simulink model "drillingRigMss"  (R2015a)
settings: Solver=ode15s  StartTime=-1500  StopTime=1445  FixedStep=1e-3  RelTol=1e-6
values from neighbouring files (symbols this model uses):
  busTieOpens = 200    [initDrillingRigMSStoolbox.m]
  connectedGensets = [ones(1,engines-1) zeros(1,1)].'    [initDrillingRigMSStoolbox.m]
  connectedGensetsAfter = [ones(1,engines-2) zeros(1,2)].'    [initDrillingRigMSStoolbox.m]
  connectedGensetsSwitchTime = busTieOpens+50    (= 250)    [initDrillingRigMSStoolbox.m]
  connectedThrusters = [ones(1,nThrusters-0) zeros(1,0)].'    [initDrillingRigMSStoolbox.m]
  connectedThrustersAfter = [ones(1,nThrusters-1) zeros(1,1)].'    [initDrillingRigMSStoolbox.m]
  connectedThrustersSwitchTime = connectedGensetsSwitchTime+2    (= 252)    [initDrillingRigMSStoolbox.m]
  dAngleCost = 20    [initDrillingRigMSStoolbox.m]
  dfCost = 1    [initDrillingRigMSStoolbox.m]
  engines = 6    [initDrillingRigMSStoolbox.m]
  nSwitchboard = 3    [initDrillingRigMSStoolbox.m]
  nThrusters = 6    [initDrillingRigMSStoolbox.m]
  pmsSamplingTime = .1    (= 0.1)    [initDrillingRigMSStoolbox.m]
  rampTimeUpload = 30    [initDrillingRigMSStoolbox.m]
  singularityAvoidanceCostGain = .1    (= 0.1)    [initDrillingRigMSStoolbox.m]
  singularityAvoidanceCostSmoother = .0001    (= 0.0001)    [initDrillingRigMSStoolbox.m]
  thrustAllocationSamplingTime = 1    [initDrillingRigMSStoolbox.m]
  u_c = [-1 ... (first row only)    [initDrillingRigMSStoolbox.m]
  useObserver = 1    [initDrillingRigMSStoolbox.m]
  vNL0 = voltageNoQLoad*ones(engines,1)    [initDrillingRigMSStoolbox.m]
  waveForceAmplitude = 1*waveFrequency^2*.2*(vessel.MA(1,1)+vessel.MA(1,1))*[1;0;0]    [initDrillingRigMSStoolbox.m]
  waveFrequency = .3*2*pi    (= 1.88495559215)    [initDrillingRigMSStoolbox.m]
  windForce = D([1 2 6],[1 2 6])*u_c*1    [initDrillingRigMSStoolbox.m]
  wNL0 = 1./(1-Droop*.5)    [initDrillingRigMSStoolbox.m]
  x_ref = [0; 0; 0]    [initDrillingRigMSStoolbox.m]
undefined symbols (not defined in the file or in its folder): dp, generators, observer, TA_sampling_time, thrusters
undefined symbols (not defined in the file): vessel
libraries: genset x6, switchboard x6, thrusterLib x6, LoadOthers x3, simulink x2, pms x1, marine_gnc x1
settings Model: Creator=torstebo  LastModifiedBy=torstebo
settings SolverCC: SolverJacobianMethodControl=FullPerturbation
settings DataIOCC: Decimation=10  InitialState=xFinal  LimitDataPoints=off  LoadInitialState=on  SaveFinalState=on  SaveCompleteFinalSimState=on  SaveFormat=StructureWithTime  SaveOutput=off  DSMLogging=off  InspectSignalLogs=on  SaveTime=off
settings OptimizationCC: AccelVerboseBuild=on
settings DebuggingCC: UnderspecifiedInitializationDetection=Classic  MergeDetectMultiDrivingBlocksExec=none  SolverPrmCheckMsg=warning  StateNameClashWarn=warning

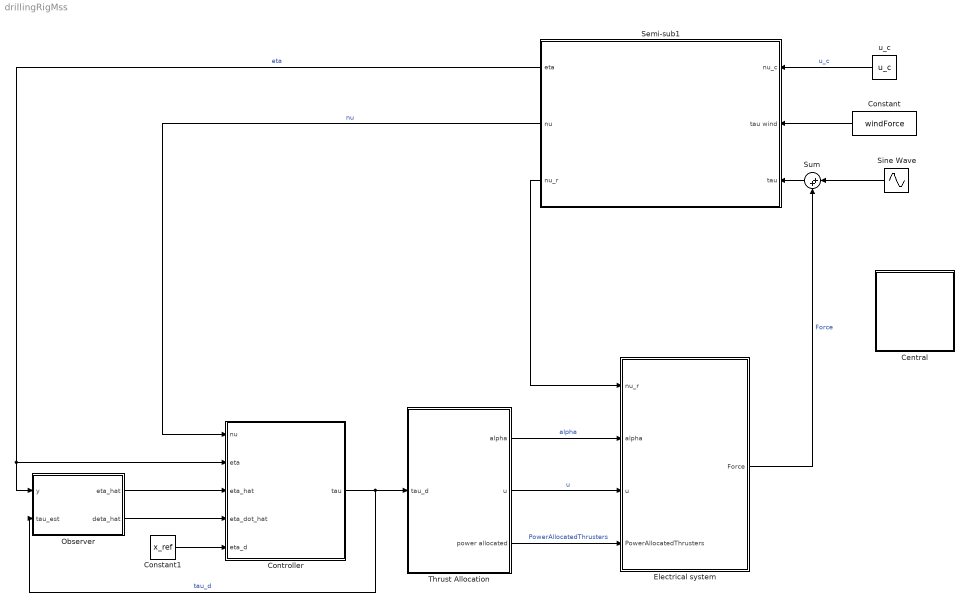
== system drillingRigMss ==
  Central : Subsystem
  Constant : Constant  Value=windForce
  Constant1 : Constant  Value=x_ref
  Controller : Subsystem
  Electrical system : Subsystem  Tag=electricSystem
  Observer : Subsystem
  Semi-sub1 : Subsystem  InitFcn=load MDGmodels/rig  mask(Semi-submersiblel (6 DOF)){D=vessel.D, G=vessel.G, MA=vessel.MA, MRB=vessel.MRB}
      mask prompts: D "Linear damping matrix: D"; G "Spring matrix G:"; MA "System inertia added mass matrix: M"; MRB "System inertia rigid-body matrix"
      mask help:
      | Semi-submersible low-speed model for DP.
      |
      | Inputs:
      |
      |    tau = 6 DOF control input vector (generalized force)
      |
      | Outputs:
      |
      |    eta = [x, y, z, phi, theta, psi]'
      |    nu  = [u, v, w, p, q, r]'
      mask Display:
      | image(imread('figs/semisub.jpg'))
      | color('white'); port_label('output', 1, 'eta')
      | color('white'); port_label('output', 2, 'nu')
      | color('white'); port_label('output', 3, 'nu_r')
      | color('white'); port_label('input', 1, 'nu_c')
      | color('white'); port_label('input', 2, 'tau wind')
      | color('white'); port_label('input', 3, 'tau')
  Sine Wave : Sin  Amplitude=waveForceAmplitude  Frequency=waveFrequency  SampleTime=0
  Sum : Sum  Inputs=|++
  Thrust Allocation : Subsystem  SystemSampleTime=TA_sampling_time
  u_c : Constant  Value=u_c
  wires:
  u_c/1 -> Semi-sub1/1(nu_c)  "u_c"
  Constant/1 -> Semi-sub1/2(tau wind)
  Semi-sub1/1(eta) -> Controller/2(eta), Observer/1(y)  "eta"
  Electrical system/1(Force) -> Sum/2  "Force"
  Controller/1(tau) -> Observer/2(tau_est), Thrust Allocation/1(tau_d)  "tau_d"
  Thrust Allocation/1(alpha) -> Electrical system/2(alpha)  "alpha"
  Thrust Allocation/2(u) -> Electrical system/3(u)  "u"
  Semi-sub1/3(nu_r) -> Electrical system/1(nu_r)
  Thrust Allocation/3(power allocated) -> Electrical system/4(PowerAllocatedThrusters)  "PowerAllocatedThrusters"
  Constant1/1 -> Controller/5(eta_d)
  Observer/2(deta_hat) -> Controller/4(eta_dot_hat)
  Observer/1(eta_hat) -> Controller/3(eta_hat)
  Sum/1 -> Semi-sub1/3(tau)
  Sine Wave/1 -> Sum/1
  Semi-sub1/2(nu) -> Controller/1(nu)  "nu"

== system drillingRigMss/Central ==
  Electric voltage calculations : Subsystem
  Event generator : Subsystem
  Power Management System : Subsystem  Tag=PowerManagementSystem

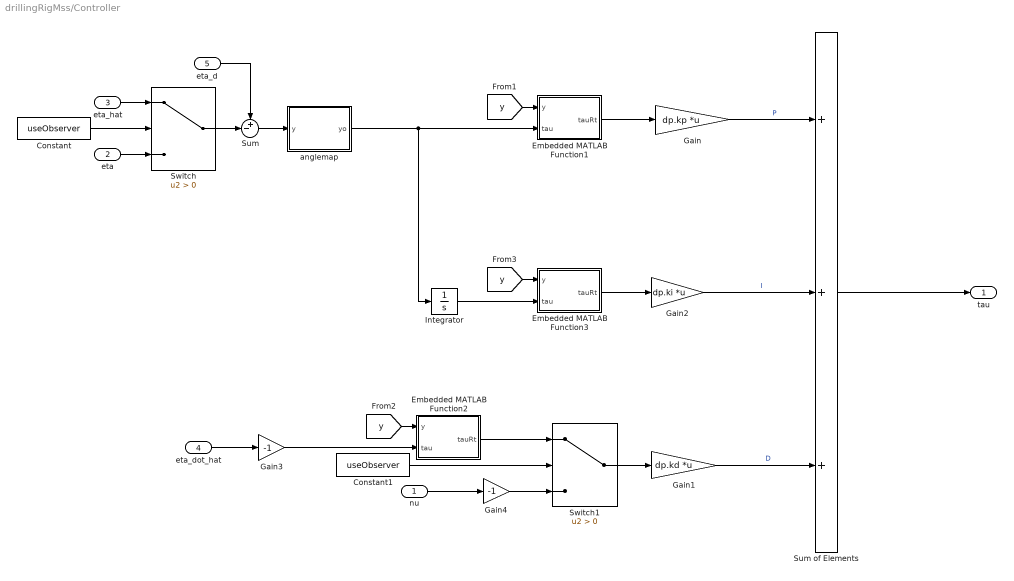
== system drillingRigMss/Controller ==
  nu : Inport
  eta : Inport  Port=2
  eta_hat : Inport  Port=3
  eta_dot_hat : Inport  Port=4
  eta_d : Inport  Port=5
  Constant : Constant  Value=useObserver
  Constant1 : Constant  Value=useObserver
  Embedded MATLAB Function1 : MATLAB Function  TreatAsAtomicUnit=on
  Embedded MATLAB Function2 : MATLAB Function  TreatAsAtomicUnit=on
  Embedded MATLAB Function3 : MATLAB Function  TreatAsAtomicUnit=on
  Gain : Gain  Gain=dp.kp  Multiplication=Matrix(K*u)
  Gain1 : Gain  Gain=dp.kd  Multiplication=Matrix(K*u)
  Gain2 : Gain  Gain=dp.ki  Multiplication=Matrix(K*u)
  Gain3 : Gain  Gain=-1
  Gain4 : Gain  Gain=-1
  Integrator : Integrator  InitialCondition=dp.ki\dp.tau0
  Sum : Sum  Inputs=+-|
  Sum of Elements : Sum  Inputs=3
  Switch : Switch  Criteria=u2 > Threshold
  Switch1 : Switch  Criteria=u2 > Threshold
  anglemap : MATLAB Function  TreatAsAtomicUnit=on
  tau : Outport
  wires:
  eta_d/1 -> Sum/1
  Gain1/1 -> Sum of Elements/3  "D"
  Sum of Elements/1 -> tau/1
  Sum/1 -> anglemap/1(y)
  [y] -> Embedded MATLAB Function1/1(y)
  Embedded MATLAB Function1/1(tauRt) -> Gain/1
  [y] -> Embedded MATLAB Function2/1(y)
  eta_dot_hat/1 -> Gain3/1
  Switch1/1 -> Gain1/1
  [y] -> Embedded MATLAB Function3/1(y)
  Integrator/1 -> Embedded MATLAB Function3/2(tau)
  Embedded MATLAB Function3/1(tauRt) -> Gain2/1
  Gain2/1 -> Sum of Elements/2  "I"
  Gain/1 -> Sum of Elements/1  "P"
  anglemap/1(yo) -> Embedded MATLAB Function1/2(tau), Integrator/1
  Gain3/1 -> Embedded MATLAB Function2/2(tau)
  nu/1 -> Gain4/1
  eta/1 -> Switch/3
  eta_hat/1 -> Switch/1
  Switch/1 -> Sum/2
  Constant/1 -> Switch/2
  Constant1/1 -> Switch1/2
  Embedded MATLAB Function2/1(tauRt) -> Switch1/1
  Gain4/1 -> Switch1/3

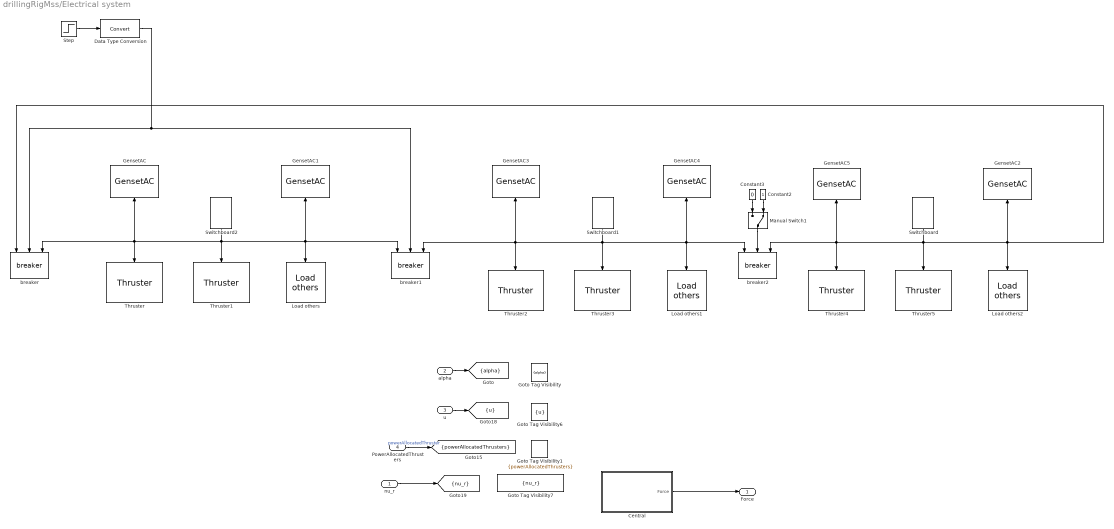
== system drillingRigMss/Electrical system ==
  nu_r : Inport  OutDataTypeStr=double
  alpha : Inport  Port=2  OutDataTypeStr=double
  u : Inport  Port=3  OutDataTypeStr=double
  PowerAllocatedThrusters : Inport  Port=4
  Central : Subsystem
  Constant2 : Constant  OutDataTypeStr=boolean
  Constant3 : Constant  Value=0  OutDataTypeStr=boolean
  Data Type Conversion : DataTypeConversion
  GensetAC : genset/GensetAC  Tag=GensetAC  genset=generators(1)  swbId=1
  GensetAC1 : genset/GensetAC  Tag=GensetAC  genset=generators(2)  swbId=1
  GensetAC2 : genset/GensetAC  Tag=GensetAC  genset=generators(6)  swbId=3
  GensetAC3 : genset/GensetAC  Tag=GensetAC  genset=generators(3)  swbId=2
  GensetAC4 : genset/GensetAC  Tag=GensetAC  genset=generators(4)  swbId=2
  GensetAC5 : genset/GensetAC  Tag=GensetAC  genset=generators(5)  swbId=3
  Goto Tag Visibility : GotoTagVisibility  GotoTag=alpha
  Goto Tag Visibility1 : GotoTagVisibility  GotoTag=powerAllocatedThrusters
  Goto Tag Visibility6 : GotoTagVisibility  GotoTag=u
  Goto Tag Visibility7 : GotoTagVisibility  GotoTag=nu_r
  Load others : LoadOthers/Load others  Tag=Load Others  swbId=1
  Load others1 : LoadOthers/Load others  Tag=Load Others  swbId=2
  Load others2 : LoadOthers/Load others  Tag=Load Others  swbId=3
  Manual Switch1 : ManualSwitch  CurrentSetting=0
  Step : Step  Time=busTieOpens  Before=1  After=0  SampleTime=0
  Switchboard : switchboard/Switchboard  Tag=Switchboard  swbId=3
  Switchboard1 : switchboard/Switchboard  Tag=Switchboard  swbId=2
  Switchboard2 : switchboard/Switchboard  Tag=Switchboard  swbId=1
  Thruster : thrusterLib/Thruster  Tag=Thruster  thruster=thrusters(1)  SwbId=1
      settings: AttributesFormatString=%<thruster>
  Thruster1 : thrusterLib/Thruster  Tag=Thruster  thruster=thrusters(2)  SwbId=1
      settings: AttributesFormatString=%<thruster>
  Thruster2 : thrusterLib/Thruster  Tag=Thruster  thruster=thrusters(3)  SwbId=2
      settings: AttributesFormatString=Thruster %<thruster.ID>
  Thruster3 : thrusterLib/Thruster  Tag=Thruster  thruster=thrusters(4)  SwbId=2
      settings: AttributesFormatString=Thruster %<thruster.ID>
  Thruster4 : thrusterLib/Thruster  Tag=Thruster  thruster=thrusters(5)  SwbId=3
      settings: AttributesFormatString=Thruster %<thruster.ID>
  Thruster5 : thrusterLib/Thruster  Tag=Thruster  thruster=thrusters(6)  SwbId=3
      settings: AttributesFormatString=Thruster %<thruster.ID>
  breaker : switchboard/breaker  Tag=SwitchboardBreaker  id=1
  breaker1 : switchboard/breaker  Tag=SwitchboardBreaker  id=2
  breaker2 : switchboard/breaker  Tag=SwitchboardBreaker  id=3
  Force : Outport  OutDataTypeStr=double
  tag scope: alpha=scoped, nu_r=scoped, powerAllocatedThrusters=scoped, u=scoped
  wires:
  alpha/1 -> [alpha]
  u/1 -> [u]
  nu_r/1 -> [nu_r]
  PowerAllocatedThrusters/1 -> [powerAllocatedThrusters]  "powerAllocatedThruster"
  Switchboard1/1 -> Thruster3/1, GensetAC4/1, breaker2/1, Load others1/1, GensetAC3/1, breaker1/3, Thruster2/1
  Switchboard/1 -> Thruster5/1, GensetAC2/1, breaker/1, Load others2/1, GensetAC5/1, breaker2/3, Thruster4/1
  Manual Switch1/1 -> breaker2/2
  Central/1(Force) -> Force/1
  Switchboard2/1 -> Thruster1/1, GensetAC/1, breaker/3, Thruster/1, GensetAC1/1, breaker1/1, Load others/1
  Constant2/1 -> Manual Switch1/2
  Constant3/1 -> Manual Switch1/1
  Data Type Conversion/1 -> breaker/2, breaker1/2
  Step/1 -> Data Type Conversion/1

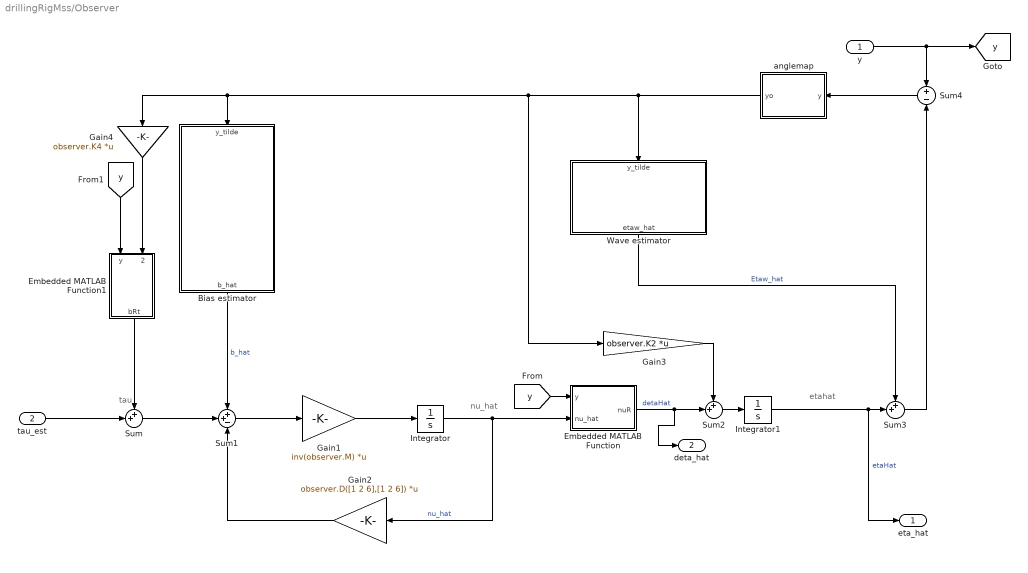
== system drillingRigMss/Observer ==
  note: nu_hat
  note: tau
  note: etahat
  y : Inport
  tau_est : Inport  Port=2
  Bias estimator : Subsystem
  Embedded MATLAB Function : MATLAB Function  TreatAsAtomicUnit=on
  Embedded MATLAB Function1 : MATLAB Function  TreatAsAtomicUnit=on
  Gain1 : Gain  Gain=inv(observer.M)  Multiplication=Matrix(K*u)
  Gain2 : Gain  Gain=observer.D([1 2 6],[1 2 6])  Multiplication=Matrix(K*u)
  Gain3 : Gain  Gain=observer.K2  Multiplication=Matrix(K*u)
  Gain4 : Gain  Gain=observer.K4  Multiplication=Matrix(K*u)
  Integrator : Integrator  InitialCondition=observer.nuHat0
  Integrator1 : Integrator  InitialCondition=observer.etaHat0
  Sum : Sum  Inputs=++|
  Sum1 : Sum  Inputs=++-
  Sum2 : Sum  Inputs=++|
  Sum3 : Sum  Inputs=++|
  Sum4 : Sum  Inputs=+-
  Wave estimator : Subsystem
  anglemap : MATLAB Function  TreatAsAtomicUnit=on
  eta_hat : Outport
  deta_hat : Outport  Port=2
  tag scope: y=global
  wires:
  tau_est/1 -> Sum/2
  Sum/1 -> Sum1/2
  Sum1/1 -> Gain1/1
  Gain1/1 -> Integrator/1
  Integrator/1 -> Gain2/1, Embedded MATLAB Function/2(nu_hat)  "nu_hat"
  Gain2/1 -> Sum1/3
  Embedded MATLAB Function/1(nuR) -> Sum2/2, deta_hat/1  "detaHat"
  Sum2/1 -> Integrator1/1
  Integrator1/1 -> Sum3/2, eta_hat/1  "etaHat"
  Sum3/1 -> Sum4/2
  y/1 -> Sum4/1, [y]
  Wave estimator/1(etaw_hat) -> Sum3/1  "Etaw_hat"
  Gain3/1 -> Sum2/1
  [y] -> Embedded MATLAB Function/1(y)
  Bias estimator/1(b_hat) -> Sum1/1  "b_hat"
  Gain4/1 -> Embedded MATLAB Function1/2(b_hat)
  [y] -> Embedded MATLAB Function1/1(y)
  Embedded MATLAB Function1/1(bRt) -> Sum/1
  Sum4/1 -> anglemap/1(y)
  anglemap/1(yo) -> Wave estimator/1(y_tilde), Gain3/1, Bias estimator/1(y_tilde), Gain4/1

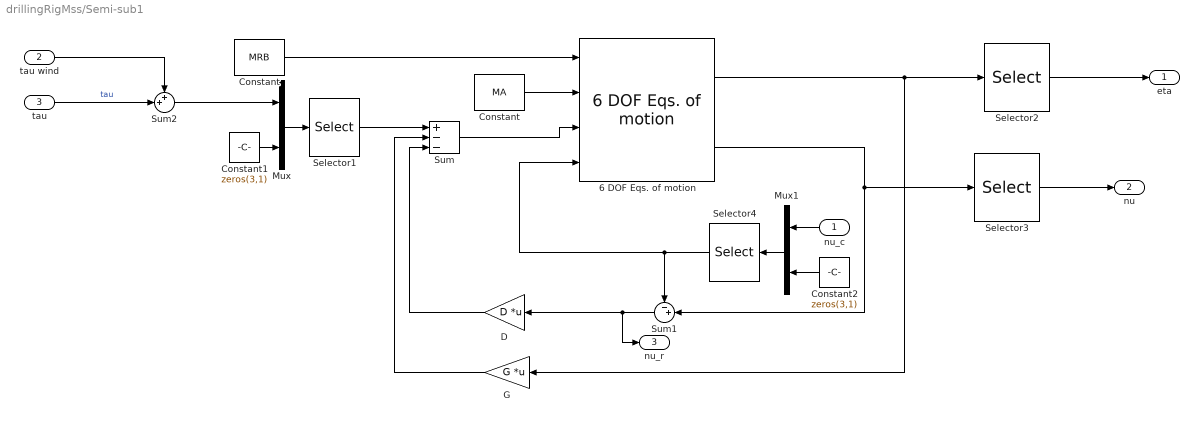
== system drillingRigMss/Semi-sub1 ==
  nu_c : Inport
  tau wind : Inport  Port=2
  tau : Inport  Port=3
  6 DOF Eqs. of motion : marine_gnc/Models/ Kinetics /6 DOF Eqs. of motion  CoriolisOnOff=on  nu0=vessel.nu0  eta0=vessel.eta0
  Constant : Constant  Value=MRB
  "Constant " : Constant  Value=MA
  Constant1 : Constant  Value=zeros(3,1)
  Constant2 : Constant  Value=zeros(3,1)
  D : Gain  Gain=D  Multiplication=Matrix(K*u)  SaturateOnIntegerOverflow=on  OutDataTypeStr=Inherit: Same as input  ParamDataTypeStr=Inherit: Same as input
  G : Gain  Gain=G  Multiplication=Matrix(K*u)  SaturateOnIntegerOverflow=on  OutDataTypeStr=Inherit: Same as input  ParamDataTypeStr=Inherit: Same as input
  Mux : Mux  Inputs=2
  Mux1 : Mux  Inputs=2
  Selector1 : Selector  InputPortWidth=6  Indices=[1 2 4 5 6 3]
  Selector2 : Selector  InputPortWidth=6  Indices=[1 2 6]
  Selector3 : Selector  InputPortWidth=6  Indices=[1 2 6]
  Selector4 : Selector  InputPortWidth=6  Indices=[1 2 4 5 6 3]
  Sum : Sum  Inputs=+--  SaturateOnIntegerOverflow=on  InputSameDT=on  OutDataTypeStr=Inherit: Same as first input
  Sum1 : Sum  Inputs=-+|  SaturateOnIntegerOverflow=on
  Sum2 : Sum  Inputs=++|
  eta : Outport  InitialOutput=0
  nu : Outport  Port=2  InitialOutput=0
  nu_r : Outport  Port=3  InitialOutput=0
  wires:
  D/1 -> Sum/3
  G/1 -> Sum/2
  6 DOF Eqs. of motion/2 -> Selector3/1, Sum1/2
  6 DOF Eqs. of motion/1 -> G/1, Selector2/1
  Constant/1 -> 6 DOF Eqs. of motion/1
  Selector4/1 -> Sum1/1, 6 DOF Eqs. of motion/4
  Sum1/1 -> nu_r/1, D/1
  Sum/1 -> 6 DOF Eqs. of motion/3
  "Constant "/1 -> 6 DOF Eqs. of motion/2
  Mux/1 -> Selector1/1
  Constant1/1 -> Mux/2
  tau/1 -> Sum2/2  "tau"
  tau wind/1 -> Sum2/1
  Sum2/1 -> Mux/1
  Selector1/1 -> Sum/1
  Selector2/1 -> eta/1
  Selector3/1 -> nu/1
  Mux1/1 -> Selector4/1
  Constant2/1 -> Mux1/2
  nu_c/1 -> Mux1/1

== system drillingRigMss/Thrust Allocation ==
  tau_d : Inport
  Constant : Constant  Value=-1
  Constant1 : Constant  Value=-1
  For Each Subsystem1 : Subsystem  TreatAsAtomicUnit=on
  From Thrusters : Subsystem  Tag=ThrusterAllocation/FromThrusters
  Subsystem : Subsystem
  Sum : Sum  Inputs=|++
  Sum1 : Sum  Inputs=|++
  Zero-Order Hold : ZeroOrderHold  SampleTime=thrustAllocationSamplingTime
  alpha : Outport
  u : Outport  Port=2
  power allocated : Outport  Port=3
  wires:
  For Each Subsystem1/11(turnTime) -> Subsystem/16(turnTime)  "turnTime"
  For Each Subsystem1/7(KT2P) -> Subsystem/12(KT2P)  "KT2P"
  For Each Subsystem1/6(Thrusters on) -> Subsystem/11(Thrusters on)  "thurstersOn"
  For Each Subsystem1/5(u_old) -> Subsystem/10(f_old)  "f"
  For Each Subsystem1/4(alpha) -> Subsystem/9(Alpha_old)  "alpha"
  For Each Subsystem1/3(Tau Max) -> Subsystem/8(Tau Max)  "tauMax"
  For Each Subsystem1/2(ThrusterPostitionY) -> Subsystem/7(Thruster Position Y)  "posY"
  For Each Subsystem1/1(ThrusterPostitionX) -> Subsystem/6(Thruster Position X)  "posX"
  [nBus] -> Subsystem/5(N bus)  "nBus"
  Sum/1 -> Subsystem/4(Switchboard to bus)  "s2b"
  tau_d/1 -> Subsystem/1(tau_d)  "tau_d"
  Constant/1 -> Sum/2
  [switchboard2bus] -> Sum/1
  From Thrusters/1(Thruster) -> Zero-Order Hold/1  "Thruster"
  Sum1/1 -> Subsystem/13(Thruster 2 Switchboard)  "t2s"
  Constant1/1 -> Sum1/2
  For Each Subsystem1/8(Thruster 2 Switchboard) -> Sum1/1
  For Each Subsystem1/9(fRampTime) -> Subsystem/14(fRampTime)  "fRampTime"
  For Each Subsystem1/10(f min) -> Subsystem/15(u min)  "fMin"
  For Each Subsystem1/12(rotable) -> Subsystem/17(rotable)  "rotable"
  For Each Subsystem1/13(reversePowerFactor) -> Subsystem/18(Reverse thrust power gain)  "reversePowerFactor"
  [FastLoadReductionThrusters] -> Subsystem/3(Fast Load Reduction Thruster)  "FLR"
  Zero-Order Hold/1 -> For Each Subsystem1/1(In1)
  [powerAvailableDP] -> Subsystem/2(Power Available Bus)  "pADP"
  Subsystem/2(U) -> u/1  "u"
  Subsystem/3(Power Allocated) -> power allocated/1
  Subsystem/1(Alpha) -> alpha/1  "alpha"

== system drillingRigMss/Central/Electric voltage calculations ==
  Busses : Subsystem
      mask Display:
      | image(imread('figs/switchboard.jpg'))
      | port_label('input',1,'Power Loads')
      | port_label('input',2,'nbus')
      | port_label('input',3,'switchboard2bus')
      | port_label('input',4,'Generators')
      | port_label('output',1,'switchboard')
  From Gensets : Subsystem  Tag=FromGeneratorsetElectric
  From breakers : Subsystem  Tag=FromBreakers
  From loads : Subsystem  Tag=FromLoads
  Switchboard2Bus : Subsystem  Tag=Switchboard2Bus  mask{nSwitchboards=3}
      mask prompts: nSwitchboards "Number of Switchboards"
  tag scope: switchboard=global
  wires:
  From breakers/1(Breakers) -> Switchboard2Bus/1(Breakers)
  From loads/1(Loads) -> Busses/1(powerLoads)
  From Gensets/1(Generators) -> Busses/4(Generatorset)
  Switchboard2Bus/2(switchboard2bus) -> Busses/3(switchboard2bus)
  Switchboard2Bus/1(nbus) -> Busses/2(nbus)
  Busses/1(switchboard bus) -> [switchboard]

== system drillingRigMss/Central/Event generator ==
  Compare To Constant : simulink/Logic and Bit Operations/Compare To Constant  relop=>  const=0  OutDataTypeStr=boolean
  Compare To Constant1 : simulink/Logic and Bit Operations/Compare To Constant  relop=>  const=0  OutDataTypeStr=boolean
  Step1 : Step  Time=connectedGensetsSwitchTime  Before=connectedGensets  After=connectedGensetsAfter  SampleTime=0
  Step2 : Step  Time=connectedThrustersSwitchTime  Before=connectedThrusters  After=connectedThrustersAfter  SampleTime=0
  tag scope: gensetsOn=global, thrustersOn=global
  wires:
  Compare To Constant1/1 -> [thrustersOn]
  Step1/1 -> Compare To Constant/1
  Compare To Constant/1 -> [gensetsOn]
  Step2/1 -> Compare To Constant1/1

== system drillingRigMss/Central/Power Management System ==
  From Batteries : Subsystem  Tag=PowerManagementSystem/FromBatteries  Commented=on
  From Generatorsets : Subsystem  Tag=PowerManagementSystem/FromGeneratorset
  From Load others : Subsystem  Tag=PowerManagementSystem/LoadOthersFrom
  From Thrusters : Subsystem  Tag=PowerManagementSystem/ThrusterFrom
  Genset Control : Subsystem
  Log Power : Subsystem
  Power Management System : pms/Subsystem  TSample=pmsSamplingTime  reactionTimePowerAvaialble=reactionTimePowerAvaialble  rampTimePowerAvaialble=rampTimePowerAvaialble  FlrRestoreTime=flrRestoreTime  FlrRampTime=flrRampTime  nSwb=nSwitchboard  nThruster=nThrusters  nBatteries=nBatteries  DPPowerAvailableBias=powerDesiredDPBias  DPPowerAvailableGain=powerDesiredDPGain  PMSenableFaultDetection=PMSenableFaultDetection
  Terminator : Terminator
  Terminator2 : Terminator
  tag scope: FastLoadReductionThrusters=global, GensetVNL=global, GensetWNL=global, powerAvailableDP=global, powerAvailableHighPriority=global, powerAvailableLowPriority=global
  wires:
  Power Management System/4 -> Log Power/2(FastLoadReductionThrusters), [FastLoadReductionThrusters]  "PowerAvailableThrusters"
  Power Management System/6 -> Log Power/4(powerAvailableHighPriority), [powerAvailableHighPriority]  "PowerAvailableHP"
  Power Management System/3 -> Log Power/1(powerAvailableDP), [powerAvailableDP]  "powerAvailableDP"
  Power Management System/5 -> Log Power/3(powerAvailableLowPriority), [powerAvailableLowPriority]  "PowerAvailableLP"
  [nBus] -> Power Management System/2
  Power Management System/1 -> Terminator2/1  "powerDP"
  Power Management System/2 -> Terminator/1  "powerDesiredDP"
  [switchboard2bus] -> Power Management System/1
  From Load others/1(PowerDesiredLowPriority) -> Power Management System/3
  From Load others/3(PowerDesiredHighPriority) -> Power Management System/5
  From Load others/2(PowerLowPriority) -> Power Management System/4
  From Load others/4(PowerHighPriority) -> Power Management System/6
  From Thrusters/1(Thruster Power) -> Power Management System/7
  From Thrusters/2(Thruster2SwbId) -> Power Management System/8
  From Thrusters/3(Thruster RatedPower) -> Power Management System/9
  From Thrusters/4(Thruster Connected) -> Power Management System/10
  From Generatorsets/1(GensetsDeliveredPower) -> Power Management System/14
  From Generatorsets/2(GensetsPowerAvailable) -> Power Management System/15
  From Generatorsets/4(GensetsRatedPower) -> Power Management System/17
  Genset Control/1(wNL) -> [GensetWNL]
  From Generatorsets/3(GensetsConnected) -> Power Management System/16
  From Generatorsets/5(GensetsSwbID) -> Genset Control/1(GensetsSwbID), Power Management System/18
  From Generatorsets/6(GensetsConnected1) -> Genset Control/2(GensetsConnected)
  Genset Control/2(vNL) -> [GensetVNL]
  From Batteries/3(BatteriesSwbId) -> Power Management System/13
  From Batteries/2(BatteriesPowerAvailable) -> Power Management System/12
  From Batteries/1(BatteriesDeliveredPower) -> Power Management System/11

== system drillingRigMss/Electrical system/Central ==
  From Force : Subsystem  Tag=ForceFrom
  Force : Outport  Tag=ForceFrom  OutDataTypeStr=double
  wires:
  From Force/1(Force) -> Force/1

== system drillingRigMss/Observer/Bias estimator ==
  y_tilde : Inport
  Embedded MATLAB Function : MATLAB Function  TreatAsAtomicUnit=on
  Gain3 : Gain  Gain=observer.K3  Multiplication=Matrix(K*u)
  Gain4 : Gain  Gain=inv(observer.T)  Multiplication=Matrix(K*u)
  Integrator1 : Integrator  InitialCondition=observer.biasForce0
  Sum1 : Sum  Inputs=+-
  b_hat : Outport
  wires:
  y_tilde/1 -> Gain3/1
  Gain3/1 -> Sum1/1
  Sum1/1 -> Integrator1/1
  Gain4/1 -> Sum1/2
  Integrator1/1 -> Gain4/1, Embedded MATLAB Function/2(b_hat)
  Embedded MATLAB Function/1(bRt) -> b_hat/1
  [y] -> Embedded MATLAB Function/1(y)

== system drillingRigMss/Observer/Wave estimator ==
  y_tilde : Inport
  Gain1 : Gain  Gain=observer.Aw  Multiplication=Matrix(K*u)
  Gain2 : Gain  Gain=observer.Cw  Multiplication=Matrix(K*u)
  Gain3 : Gain  Gain=observer.K1  Multiplication=Matrix(K*u)
  Integrator : Integrator  InitialCondition=[0 0 0 0 0 0]'
  Sum : Sum  Inputs=|++
  etaw_hat : Outport  PortDimensions=3
  wires:
  y_tilde/1 -> Gain3/1
  Gain3/1 -> Sum/1
  Sum/1 -> Integrator/1
  Integrator/1 -> Gain1/1, Gain2/1
  Gain1/1 -> Sum/2
  Gain2/1 -> etaw_hat/1

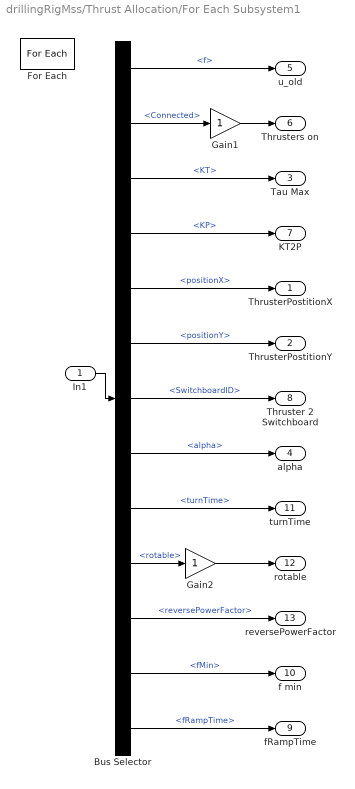
== system drillingRigMss/Thrust Allocation/For Each Subsystem1 ==
  In1 : Inport  OutDataTypeStr=Bus: ThrusterBus  Partition=on  PartitionDimension=1  PartitionWidth=1
  Bus Selector : BusSelector  OutputSignals=f,Connected,KT,KP,positionX,positionY,SwitchboardID,alpha,turnTime,rotable,reversePowerFactor,fMin,fRampTime
  For Each : ForEach  DisableCoverage=on  IndexMode=One-based
  Gain1 : Gain  OutDataTypeStr=double
  Gain2 : Gain  OutDataTypeStr=double
  ThrusterPostitionX : Outport  ConcatenationDimension=1
  ThrusterPostitionY : Outport  Port=2  ConcatenationDimension=1
  Tau Max : Outport  Port=3  ConcatenationDimension=1
  alpha : Outport  Port=4  ConcatenationDimension=1
  u_old : Outport  Port=5  ConcatenationDimension=1
  Thrusters on : Outport  Port=6  ConcatenationDimension=1
  KT2P : Outport  Port=7  ConcatenationDimension=1
  Thruster 2 Switchboard : Outport  Port=8  ConcatenationDimension=1
  fRampTime : Outport  Port=9  ConcatenationDimension=1
  f min : Outport  Port=10  ConcatenationDimension=1
  turnTime : Outport  Port=11  ConcatenationDimension=1
  rotable : Outport  Port=12  ConcatenationDimension=1
  reversePowerFactor : Outport  Port=13  ConcatenationDimension=1
  wires:
  Bus Selector/13 -> fRampTime/1  "<fRampTime>"
  Bus Selector/12 -> f min/1  "<fMin>"
  Bus Selector/11 -> reversePowerFactor/1  "<reversePowerFactor>"
  Bus Selector/9 -> turnTime/1  "<turnTime>"
  Bus Selector/10 -> Gain2/1  "<rotable>"
  Bus Selector/8 -> alpha/1  "<alpha>"
  Bus Selector/7 -> Thruster 2 Switchboard/1  "<SwitchboardID>"
  Bus Selector/6 -> ThrusterPostitionY/1  "<positionY>"
  Bus Selector/5 -> ThrusterPostitionX/1  "<positionX>"
  Gain1/1 -> Thrusters on/1
  Bus Selector/4 -> KT2P/1  "<KP>"
  Bus Selector/3 -> Tau Max/1  "<KT>"
  Bus Selector/2 -> Gain1/1  "<Connected>"
  Bus Selector/1 -> u_old/1  "<f>"
  In1/1 -> Bus Selector/1
  Gain2/1 -> rotable/1

== system drillingRigMss/Thrust Allocation/From Thrusters ==
  Vector Concatenate : Concatenate  Tag=FromThrusters/Merger  NumInputs=6
  Thruster : Outport
  wires:
  Vector Concatenate/1 -> Thruster/1
  [Thruster1] -> Vector Concatenate/1
  [Thruster2] -> Vector Concatenate/2
  [Thruster3] -> Vector Concatenate/3
  [Thruster4] -> Vector Concatenate/4
  [Thruster5] -> Vector Concatenate/5
  [Thruster6] -> Vector Concatenate/6

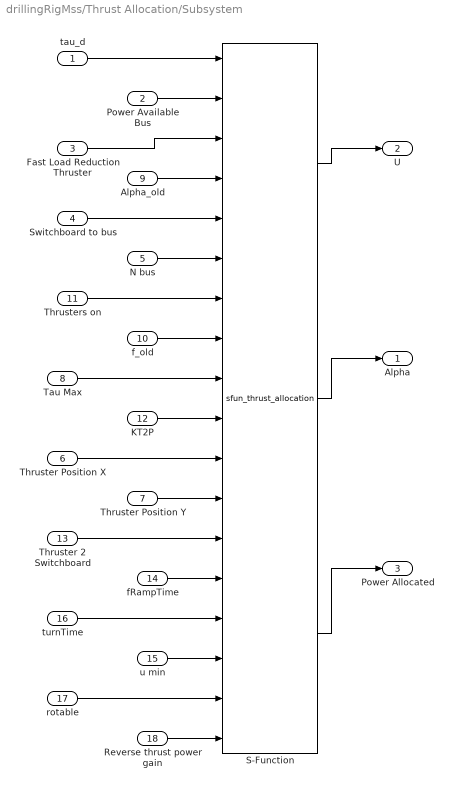
== system drillingRigMss/Thrust Allocation/Subsystem ==
  tau_d : Inport
  Power Available Bus : Inport  Port=2
  Fast Load Reduction Thruster : Inport  Port=3
  Switchboard to bus : Inport  Port=4
  N bus : Inport  Port=5
  Thruster Position X : Inport  Port=6
  Thruster Position Y : Inport  Port=7
  Tau Max : Inport  Port=8
  Alpha_old : Inport  Port=9
  f_old : Inport  Port=10
  Thrusters on : Inport  Port=11
  KT2P : Inport  Port=12
  Thruster 2 Switchboard : Inport  Port=13
  fRampTime : Inport  Port=14
  u min : Inport  Port=15
  turnTime : Inport  Port=16
  rotable : Inport  Port=17
  Reverse thrust power gain : Inport  Port=18
  S-Function : S-Function  FunctionName=sfun_thrust_allocation  Parameters=thrustAllocationSamplingTime,nThrusters,nSwitchboard,singularityAvoidanceCostGain,singularityAvoidanceCostSmoother,dfCost,dAngleCost
  Alpha : Outport
  U : Outport  Port=2
  Power Allocated : Outport  Port=3
  wires:
  f_old/1 -> S-Function/8
  Thrusters on/1 -> S-Function/7
  N bus/1 -> S-Function/6
  Switchboard to bus/1 -> S-Function/5
  Alpha_old/1 -> S-Function/4
  Fast Load Reduction Thruster/1 -> S-Function/3
  tau_d/1 -> S-Function/1
  Power Available Bus/1 -> S-Function/2
  S-Function/1 -> U/1
  S-Function/2 -> Alpha/1
  turnTime/1 -> S-Function/15
  fRampTime/1 -> S-Function/14
  Thruster 2 Switchboard/1 -> S-Function/13
  Thruster Position Y/1 -> S-Function/12
  Thruster Position X/1 -> S-Function/11
  KT2P/1 -> S-Function/10
  Tau Max/1 -> S-Function/9
  u min/1 -> S-Function/16
  S-Function/3 -> Power Allocated/1
  rotable/1 -> S-Function/17
  Reverse thrust power gain/1 -> S-Function/18

== system drillingRigMss/Central/Electric voltage calculations/Busses ==
  powerLoads : Inport  OutDataTypeStr=Bus: powerLoadsBus
  nbus : Inport  Port=2
  switchboard2bus : Inport  Port=3
  Generatorset : Inport  Port=4
  Constant2 : Constant  Value=-1
  Integrator : Integrator
  MATLAB Function1 : MATLAB Function  TreatAsAtomicUnit=on
  Merge loads : MATLAB Function  TreatAsAtomicUnit=on
  Saturation : Saturate  UpperLimit=0  LowerLimit=-1
  Sum : Sum  Inputs=++|
  Switchboard1 : MATLAB Function  TreatAsAtomicUnit=on
  Thevenin Equivalent : MATLAB Function  TreatAsAtomicUnit=on
  switchboard bus : Outport
  wires:
  Switchboard1/1(out) -> switchboard bus/1
  powerLoads/1 -> Merge loads/1(load)  "power bus"
  switchboard2bus/1 -> Switchboard1/2(switchboard2bus), Merge loads/2(swb2bus), Thevenin Equivalent/2(switchboard2bus)  "s2b"
  Generatorset/1 -> Thevenin Equivalent/3(generatorset)  "Generatorset"
  Integrator/1 -> MATLAB Function1/1(u)
  Constant2/1 -> Sum/1
  Sum/1 -> Saturation/1
  Switchboard1/2(isInputValid) -> Sum/2
  nbus/1 -> Switchboard1/3(nbus), Thevenin Equivalent/1(nbus)  "nbus"
  Merge loads/1(loads) -> Switchboard1/1(powerLoads)  "load"
  Thevenin Equivalent/1(theveninEquivalent) -> Switchboard1/4(generatorset)
  Saturation/1 -> Integrator/1

== system drillingRigMss/Central/Electric voltage calculations/From Gensets ==
  Merger : Concatenate  Tag=FromGeneratorsetElectric/Merger  NumInputs=6
  Generators : Outport
  wires:
  Merger/1 -> Generators/1
  [GeneratorsetElectric1] -> Merger/1
  [GeneratorsetElectric2] -> Merger/2
  [GeneratorsetElectric6] -> Merger/6
  [GeneratorsetElectric3] -> Merger/3
  [GeneratorsetElectric4] -> Merger/4
  [GeneratorsetElectric5] -> Merger/5

== system drillingRigMss/Central/Electric voltage calculations/From breakers ==
  MergerBreakers : Concatenate  Tag=FromBreakers/MergerBreakers  NumInputs=3
  Breakers : Outport
  wires:
  MergerBreakers/1 -> Breakers/1
  [Breaker1] -> MergerBreakers/1
  [Breaker2] -> MergerBreakers/2
  [Breaker3] -> MergerBreakers/3

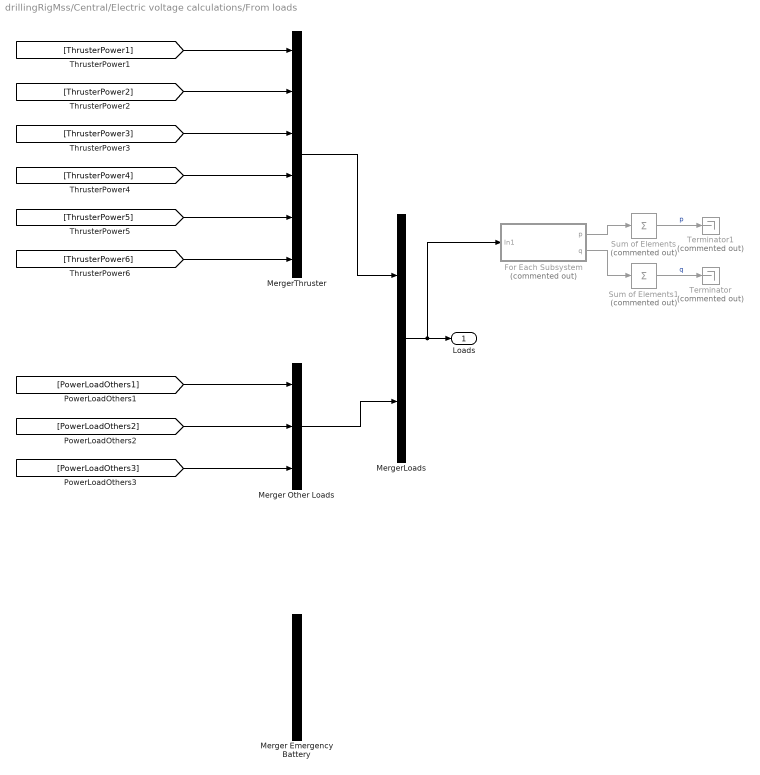
== system drillingRigMss/Central/Electric voltage calculations/From loads ==
  For Each Subsystem : Subsystem  Commented=on  TreatAsAtomicUnit=on
  Merger Emergency Battery : Concatenate  Tag=FromLoads/MergerEmergencyBattery  NumInputs=1
  Merger Other Loads : Concatenate  Tag=FromLoads/MergerOtherLoads  NumInputs=3
  MergerLoads : Concatenate  Tag=FromLoads/MergerLoads
  MergerThruster : Concatenate  Tag=FromLoads/MergerThruster  NumInputs=6
  Sum of Elements : Sum  Commented=on  Inputs=+
  Sum of Elements1 : Sum  Commented=on  Inputs=+
  Terminator : Terminator  Commented=on
  Terminator1 : Terminator  Commented=on
  Loads : Outport
  wires:
  MergerThruster/1 -> MergerLoads/1
  Merger Other Loads/1 -> MergerLoads/2
  MergerLoads/1 -> For Each Subsystem/1(In1), Loads/1
  For Each Subsystem/1(p) -> Sum of Elements/1
  For Each Subsystem/2(q) -> Sum of Elements1/1
  Sum of Elements1/1 -> Terminator/1  "q"
  Sum of Elements/1 -> Terminator1/1  "p"
  [PowerLoadOthers1] -> Merger Other Loads/1
  [PowerLoadOthers2] -> Merger Other Loads/2
  [PowerLoadOthers3] -> Merger Other Loads/3
  [ThrusterPower1] -> MergerThruster/1
  [ThrusterPower2] -> MergerThruster/2
  [ThrusterPower3] -> MergerThruster/3
  [ThrusterPower4] -> MergerThruster/4
  [ThrusterPower5] -> MergerThruster/5
  [ThrusterPower6] -> MergerThruster/6

== system drillingRigMss/Central/Electric voltage calculations/Switchboard2Bus ==
  Breakers : Inport
  MATLAB Function : MATLAB Function  TreatAsAtomicUnit=on
  nbus : Outport
  switchboard2bus : Outport  Port=2
  tag scope: nBus=global, switchboard2bus=global
  wires:
  MATLAB Function/2(switchboard2bus) -> switchboard2bus/1, [switchboard2bus]
  MATLAB Function/1(nbus) -> nbus/1, [nBus]
  Breakers/1 -> MATLAB Function/1(breaker)

== system drillingRigMss/Central/Power Management System/From Batteries ==
  For Each Subsystem : Subsystem  TreatAsAtomicUnit=on
  Vector Concatenate : Concatenate  Tag=PowerManagementSystem/FromBatteries/Merger  NumInputs=1
  Zero-Order Hold : ZeroOrderHold  SampleTime=pmsSamplingTime
  BatteriesDeliveredPower : Outport
  BatteriesPowerAvailable : Outport  Port=2
  BatteriesSwbId : Outport  Port=3
  wires:
  For Each Subsystem/3(switchboardId) -> BatteriesSwbId/1
  For Each Subsystem/2(powerAvailable) -> BatteriesPowerAvailable/1
  For Each Subsystem/1(powerDelivered) -> BatteriesDeliveredPower/1
  Vector Concatenate/1 -> Zero-Order Hold/1
  Zero-Order Hold/1 -> For Each Subsystem/1(In1)
  [EmergencyBattery1] -> Vector Concatenate/1

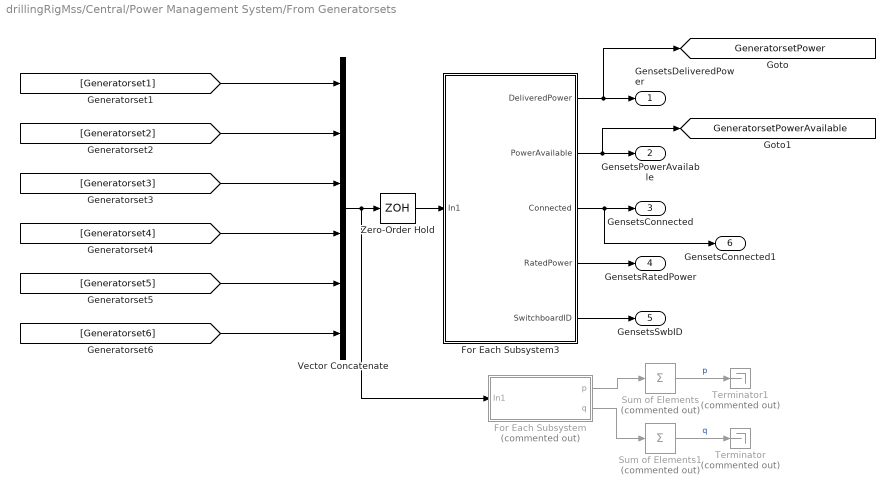
== system drillingRigMss/Central/Power Management System/From Generatorsets ==
  For Each Subsystem : Subsystem  Commented=on  TreatAsAtomicUnit=on
  For Each Subsystem3 : Subsystem  TreatAsAtomicUnit=on
  Sum of Elements : Sum  Commented=on  Inputs=+
  Sum of Elements1 : Sum  Commented=on  Inputs=+
  Terminator : Terminator  Commented=on
  Terminator1 : Terminator  Commented=on
  Vector Concatenate : Concatenate  Tag=PowerManagementSystem/FromGeneratorset/Merger  NumInputs=6
  Zero-Order Hold : ZeroOrderHold  SampleTime=pmsSamplingTime
  GensetsDeliveredPower : Outport  OutDataTypeStr=double
  GensetsPowerAvailable : Outport  Port=2  OutDataTypeStr=double
  GensetsConnected : Outport  Port=3  OutDataTypeStr=boolean
  GensetsRatedPower : Outport  Port=4  OutDataTypeStr=double
  GensetsSwbID : Outport  Port=5  OutDataTypeStr=uint8
  GensetsConnected1 : Outport  Port=6  OutDataTypeStr=boolean
  tag scope: GeneratorsetPower=global, GeneratorsetPowerAvailable=global
  wires:
  For Each Subsystem3/3(Connected) -> GensetsConnected1/1, GensetsConnected/1
  For Each Subsystem3/5(SwitchboardID) -> GensetsSwbID/1
  For Each Subsystem3/2(PowerAvailable) -> [GeneratorsetPowerAvailable], GensetsPowerAvailable/1
  For Each Subsystem3/4(RatedPower) -> GensetsRatedPower/1
  For Each Subsystem3/1(DeliveredPower) -> [GeneratorsetPower], GensetsDeliveredPower/1
  Vector Concatenate/1 -> Zero-Order Hold/1, For Each Subsystem/1(In1)
  For Each Subsystem/1(p) -> Sum of Elements/1
  For Each Subsystem/2(q) -> Sum of Elements1/1
  Sum of Elements1/1 -> Terminator/1  "q"
  Sum of Elements/1 -> Terminator1/1  "p"
  Zero-Order Hold/1 -> For Each Subsystem3/1(In1)
  [Generatorset1] -> Vector Concatenate/1
  [Generatorset2] -> Vector Concatenate/2
  [Generatorset6] -> Vector Concatenate/6
  [Generatorset3] -> Vector Concatenate/3
  [Generatorset4] -> Vector Concatenate/4
  [Generatorset5] -> Vector Concatenate/5

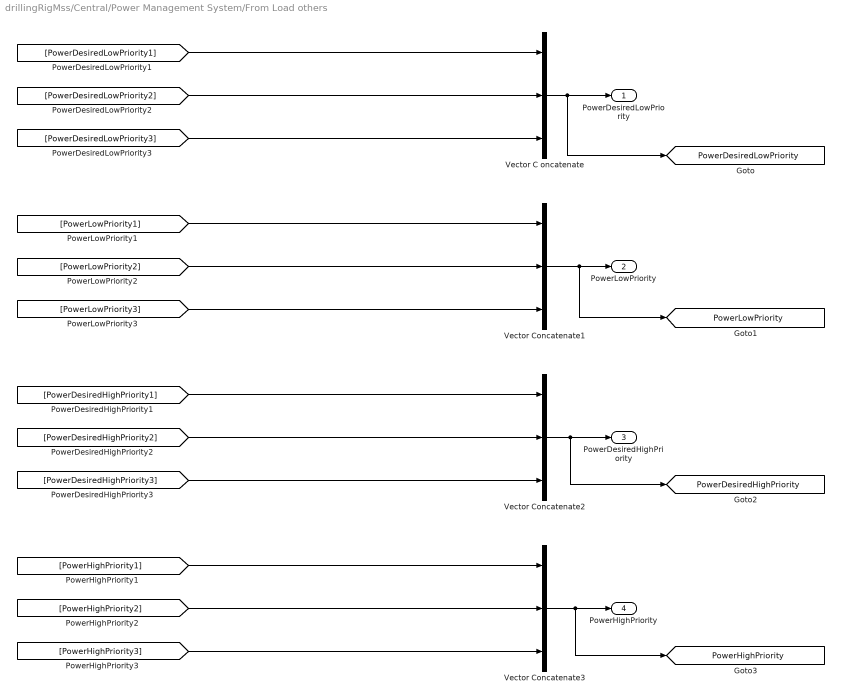
== system drillingRigMss/Central/Power Management System/From Load others ==
  Vector C oncatenate : Concatenate  Tag=PowerManagementSystem/LoadOthersFrom/PowerDesiredLowPriority  NumInputs=3
  Vector Concatenate1 : Concatenate  Tag=PowerManagementSystem/LoadOthersFrom/PowerLowPriority  NumInputs=3
  Vector Concatenate2 : Concatenate  Tag=PowerManagementSystem/LoadOthersFrom/PowerDesiredHighPriority  NumInputs=3
  Vector Concatenate3 : Concatenate  Tag=PowerManagementSystem/LoadOthersFrom/PowerHighPriority  NumInputs=3
  PowerDesiredLowPriority : Outport
  PowerLowPriority : Outport  Port=2
  PowerDesiredHighPriority : Outport  Port=3
  PowerHighPriority : Outport  Port=4
  tag scope: PowerDesiredHighPriority=global, PowerDesiredLowPriority=global, PowerHighPriority=global, PowerLowPriority=global
  wires:
  Vector C oncatenate/1 -> PowerDesiredLowPriority/1, [PowerDesiredLowPriority]
  Vector Concatenate1/1 -> [PowerLowPriority], PowerLowPriority/1
  Vector Concatenate2/1 -> [PowerDesiredHighPriority], PowerDesiredHighPriority/1
  Vector Concatenate3/1 -> [PowerHighPriority], PowerHighPriority/1
  [PowerDesiredLowPriority1] -> Vector C oncatenate/1
  [PowerLowPriority1] -> Vector Concatenate1/1
  [PowerDesiredHighPriority1] -> Vector Concatenate2/1
  [PowerHighPriority1] -> Vector Concatenate3/1
  [PowerDesiredLowPriority2] -> Vector C oncatenate/2
  [PowerLowPriority2] -> Vector Concatenate1/2
  [PowerDesiredHighPriority2] -> Vector Concatenate2/2
  [PowerHighPriority2] -> Vector Concatenate3/2
  [PowerDesiredLowPriority3] -> Vector C oncatenate/3
  [PowerLowPriority3] -> Vector Concatenate1/3
  [PowerDesiredHighPriority3] -> Vector Concatenate2/3
  [PowerHighPriority3] -> Vector Concatenate3/3

== system drillingRigMss/Central/Power Management System/From Thrusters ==
  For Each Subsystem : Subsystem  TreatAsAtomicUnit=on
  Vector Concatenate : Concatenate  Tag=FromThrusters/Merger  NumInputs=6
  Zero-Order Hold : ZeroOrderHold  SampleTime=pmsSamplingTime
  Thruster Power : Outport
  Thruster2SwbId : Outport  Port=2
  Thruster RatedPower : Outport  Port=3
  Thruster Connected : Outport  Port=4
  tag scope: ThrusterPower=global
  wires:
  For Each Subsystem/3(RatedPower) -> Thruster RatedPower/1
  For Each Subsystem/2(switchboardId) -> Thruster2SwbId/1
  For Each Subsystem/1(power) -> [ThrusterPower], Thruster Power/1
  For Each Subsystem/4(Connected) -> Thruster Connected/1
  Vector Concatenate/1 -> Zero-Order Hold/1
  Zero-Order Hold/1 -> For Each Subsystem/1(In1)
  [Thruster1] -> Vector Concatenate/1
  [Thruster2] -> Vector Concatenate/2
  [Thruster3] -> Vector Concatenate/3
  [Thruster4] -> Vector Concatenate/4
  [Thruster5] -> Vector Concatenate/5
  [Thruster6] -> Vector Concatenate/6

== system drillingRigMss/Central/Power Management System/Genset Control ==
  GensetsSwbID : Inport
  GensetsConnected : Inport  Port=2
  Clock : Clock
  MATLAB Function : MATLAB Function  TreatAsAtomicUnit=on
  wNL : Outport
  vNL : Outport  Port=2
  wires:
  MATLAB Function/1(wNL) -> wNL/1
  [switchboard] -> MATLAB Function/2(switchboard)
  GensetsConnected/1 -> MATLAB Function/1(gensetConnected)
  GensetsSwbID/1 -> MATLAB Function/3(gensetSwbId)
  Clock/1 -> MATLAB Function/4(time)
  MATLAB Function/2(vNL) -> vNL/1

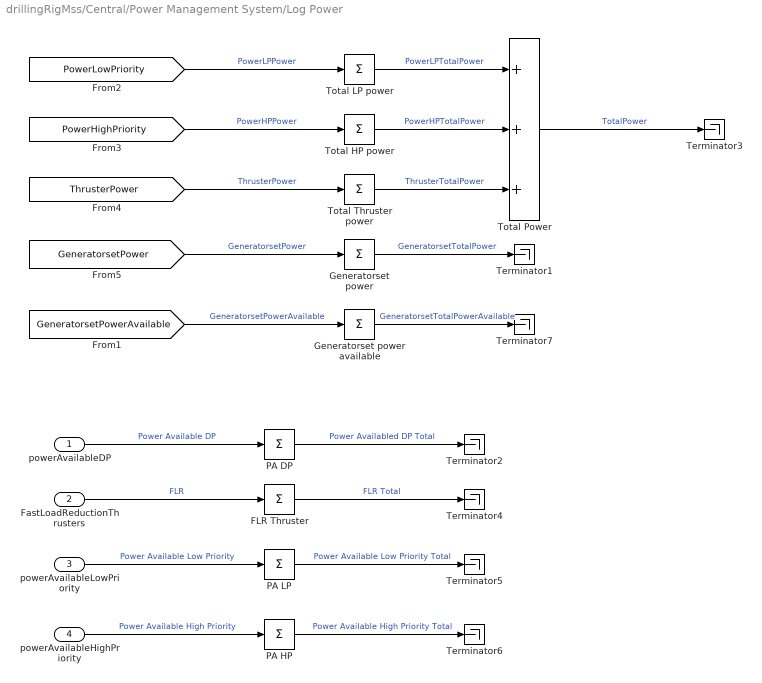
== system drillingRigMss/Central/Power Management System/Log Power ==
  powerAvailableDP : Inport
  FastLoadReductionThrusters : Inport  Port=2
  powerAvailableLowPriority : Inport  Port=3
  powerAvailableHighPriority : Inport  Port=4
  FLR Thruster : Sum  Inputs=+
  Generatorset power : Sum  Inputs=+
  Generatorset power available : Sum  Inputs=+
  PA DP : Sum  Inputs=+
  PA HP : Sum  Inputs=+
  PA LP : Sum  Inputs=+
  Terminator{1..7} (7 alike) : Terminator
  Total HP power : Sum  Inputs=+
  Total LP power : Sum  Inputs=+
  Total Power : Sum  Inputs=3
  Total Thruster power : Sum  Inputs=+
  wires:
  [PowerHighPriority] -> Total HP power/1  "PowerHPPower"
  Total HP power/1 -> Total Power/2  "PowerHPTotalPower"
  Total Power/1 -> Terminator3/1  "TotalPower"
  Generatorset power/1 -> Terminator1/1  "GeneratorsetTotalPower"
  [GeneratorsetPower] -> Generatorset power/1  "GeneratorsetPower"
  [ThrusterPower] -> Total Thruster power/1  "ThrusterPower"
  Total Thruster power/1 -> Total Power/3  "ThrusterTotalPower"
  Total LP power/1 -> Total Power/1  "PowerLPTotalPower"
  [PowerLowPriority] -> Total LP power/1  "PowerLPPower"
  powerAvailableDP/1 -> PA DP/1  "Power Available DP"
  PA DP/1 -> Terminator2/1  "Power Availabled DP Total"
  FastLoadReductionThrusters/1 -> FLR Thruster/1  "FLR"
  FLR Thruster/1 -> Terminator4/1  "FLR Total"
  powerAvailableLowPriority/1 -> PA LP/1  "Power Available Low Priority"
  powerAvailableHighPriority/1 -> PA HP/1  "Power Available High Priority"
  PA LP/1 -> Terminator5/1  "Power Available Low Priority Total"
  PA HP/1 -> Terminator6/1  "Power Available High Priority Total"
  Generatorset power available/1 -> Terminator7/1  "GeneratorsetTotalPowerAvailable"
  [GeneratorsetPowerAvailable] -> Generatorset power available/1  "GeneratorsetPowerAvailable"

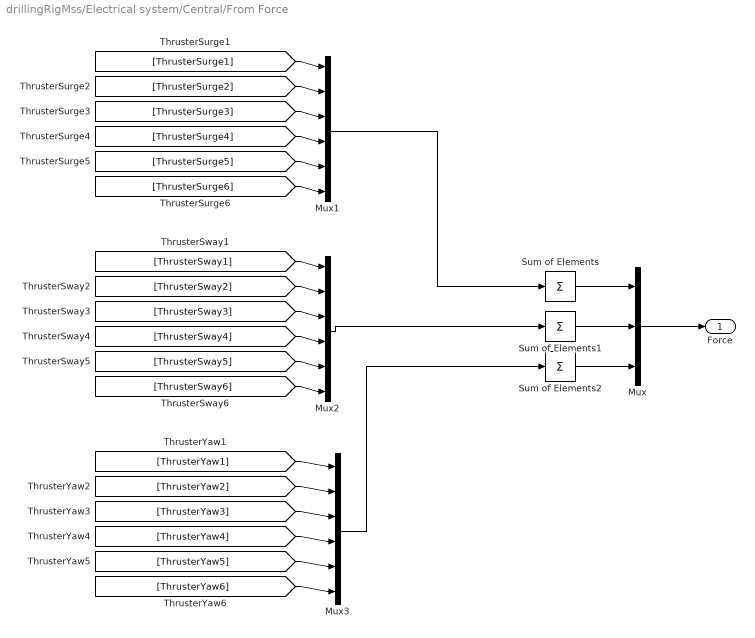
== system drillingRigMss/Electrical system/Central/From Force ==
  Mux : Mux  Inputs=3
  Mux1 : Mux  Tag=ForceFrom/SurgeMerger  Inputs=6
  Mux2 : Mux  Tag=ForceFrom/SwayMerger  Inputs=6
  Mux3 : Mux  Tag=ForceFrom/YawMerger  Inputs=6
  Sum of Elements : Sum  Inputs=+
  Sum of Elements1 : Sum  Inputs=+
  Sum of Elements2 : Sum  Inputs=+
  Force : Outport
  wires:
  Sum of Elements2/1 -> Mux/3
  Sum of Elements/1 -> Mux/1
  Sum of Elements1/1 -> Mux/2
  Mux/1 -> Force/1
  Mux1/1 -> Sum of Elements/1
  Mux2/1 -> Sum of Elements1/1
  Mux3/1 -> Sum of Elements2/1
  [ThrusterSurge1] -> Mux1/1
  [ThrusterSway1] -> Mux2/1
  [ThrusterYaw1] -> Mux3/1
  [ThrusterSurge2] -> Mux1/2
  [ThrusterSway2] -> Mux2/2
  [ThrusterYaw2] -> Mux3/2
  [ThrusterSurge3] -> Mux1/3
  [ThrusterSway3] -> Mux2/3
  [ThrusterYaw3] -> Mux3/3
  [ThrusterSurge4] -> Mux1/4
  [ThrusterSway4] -> Mux2/4
  [ThrusterYaw4] -> Mux3/4
  [ThrusterSurge5] -> Mux1/5
  [ThrusterSway5] -> Mux2/5
  [ThrusterYaw5] -> Mux3/5
  [ThrusterSurge6] -> Mux1/6
  [ThrusterSway6] -> Mux2/6
  [ThrusterYaw6] -> Mux3/6

== system drillingRigMss/Central/Electric voltage calculations/From loads/For Each Subsystem ==
  In1 : Inport  Partition=on  PartitionDimension=1  PartitionWidth=1
  Bus Selector : BusSelector  OutputSignals=p,q
  For Each : ForEach  DisableCoverage=on  IndexMode=One-based
  p : Outport  ConcatenationDimension=1
  q : Outport  Port=2  ConcatenationDimension=1
  wires:
  In1/1 -> Bus Selector/1
  Bus Selector/1 -> p/1  "<p>"
  Bus Selector/2 -> q/1  "<q>"

== system drillingRigMss/Central/Power Management System/From Batteries/For Each Subsystem ==
  In1 : Inport  Partition=on  PartitionDimension=1  PartitionWidth=1
  Bus Selector : BusSelector  OutputSignals=powerDelivered,powerAvailable,swbId
  For Each : ForEach  DisableCoverage=on  IndexMode=One-based
  powerDelivered : Outport  OutDataTypeStr=double  ConcatenationDimension=1
  powerAvailable : Outport  Port=2  OutDataTypeStr=double  ConcatenationDimension=1
  switchboardId : Outport  Port=3  OutDataTypeStr=uint8  ConcatenationDimension=1
  wires:
  In1/1 -> Bus Selector/1
  Bus Selector/1 -> powerDelivered/1  "<powerDelivered>"
  Bus Selector/2 -> powerAvailable/1  "<powerAvailable>"
  Bus Selector/3 -> switchboardId/1  "<swbId>"

== system drillingRigMss/Central/Power Management System/From Generatorsets/For Each Subsystem ==
  In1 : Inport  Partition=on  PartitionDimension=1  PartitionWidth=1
  Bus Selector : BusSelector  OutputSignals=P,Q
  For Each : ForEach  DisableCoverage=on  IndexMode=One-based
  p : Outport  ConcatenationDimension=1
  q : Outport  Port=2  ConcatenationDimension=1
  wires:
  In1/1 -> Bus Selector/1
  Bus Selector/1 -> p/1  "<P>"
  Bus Selector/2 -> q/1  "<Q>"

== system drillingRigMss/Central/Power Management System/From Generatorsets/For Each Subsystem3 ==
  In1 : Inport  OutDataTypeStr=Bus: Genset2PMS  Partition=on  PartitionDimension=1  PartitionWidth=1
  Bus Selector : BusSelector  OutputSignals=SwitchboardID,Sb,P,Connected,powerAvailable
  For Each : ForEach  DisableCoverage=on  IndexMode=One-based
  DeliveredPower : Outport  OutDataTypeStr=double  ConcatenationDimension=1
  PowerAvailable : Outport  Port=2  OutDataTypeStr=double  ConcatenationDimension=1
  Connected : Outport  Port=3  OutDataTypeStr=boolean  ConcatenationDimension=1
  RatedPower : Outport  Port=4  OutDataTypeStr=double  ConcatenationDimension=1
  SwitchboardID : Outport  Port=5  OutDataTypeStr=uint8  ConcatenationDimension=1
  wires:
  In1/1 -> Bus Selector/1
  Bus Selector/2 -> RatedPower/1  "<Sb>"
  Bus Selector/1 -> SwitchboardID/1  "<SwitchboardID>"
  Bus Selector/3 -> DeliveredPower/1  "<P>"
  Bus Selector/4 -> Connected/1  "<Connected>"
  Bus Selector/5 -> PowerAvailable/1  "<powerAvailable>"

== system drillingRigMss/Central/Power Management System/From Thrusters/For Each Subsystem ==
  In1 : Inport  OutDataTypeStr=Bus: ThrusterBus  Partition=on  PartitionDimension=1  PartitionWidth=1
  Bus Selector : BusSelector  OutputSignals=power.p,SwitchboardID,Connected,powerMax
  For Each : ForEach  DisableCoverage=on  IndexMode=One-based
  power : Outport  OutDataTypeStr=double  ConcatenationDimension=1
  switchboardId : Outport  Port=2  OutDataTypeStr=uint8  ConcatenationDimension=1
  RatedPower : Outport  Port=3  OutDataTypeStr=double  ConcatenationDimension=1
  Connected : Outport  Port=4  OutDataTypeStr=boolean  ConcatenationDimension=1
  wires:
  In1/1 -> Bus Selector/1
  Bus Selector/1 -> power/1  "<p>"
  Bus Selector/2 -> switchboardId/1  "<SwitchboardID>"
  Bus Selector/3 -> Connected/1  "<Connected>"
  Bus Selector/4 -> RatedPower/1  "<powerMax>"

== matlab function drillingRigMss/Central/Electric voltage calculations/Busses/Switchboard1 ==
  data: powerLoads input; out output Bus: swb; isInputValid output size=1; switchboard2bus input; nbus input; generatorset input
function [out, isInputValid]= switchboard(powerLoads,switchboard2bus,nbus,generatorset)
%#codegen

[out, isInputValid]= switchboardCentral(powerLoads,switchboard2bus,nbus,generatorset);

== matlab function drillingRigMss/Central/Electric voltage calculations/Busses/MATLAB Function1 ==
  data: u input
function stopper(u)
%#codegen
if ( u < -1)
    error('Bus voltage calculations have been invalid for 1 second, stopping stimulation');
end

== matlab function drillingRigMss/Central/Power Management System/Genset Control/MATLAB Function ==
  data: wNL0 parameter; vNL0 parameter; wNL output double; engines parameter; gensetConnected input; switchboard input; gensetSwbId input; time input; rampTimeUpload parameter; vNL output
function [wNL, vNL] = loadSharingControl(wNL0,vNL0,engines,gensetConnected,switchboard,gensetSwbId,time,rampTimeUpload)
wNL = ones(engines,1);
vNL = ones(engines,1);
persistent timeConnected;
if isempty(timeConnected)
    timeConnected = -inf*ones(engines,1);
end

for i = 1:engines
    if (gensetConnected(i))
        if (timeConnected(i)+rampTimeUpload<=time)
            wNL(i) = wNL0(i);
            vNL(i) = vNL0(i);
        else
            a = (time-timeConnected(i))/rampTimeUpload;
            wNL(i) = wNL0(i)*a+switchboard(gensetSwbId(i)).omega*(1-a);
            vNL(i) = vNL0(i)*a+abs(switchboard(gensetSwbId(i)).voltage)*(1-a);
    
        end
    else
        timeConnected(i) = time;
        wNL(i) = switchboard(gensetSwbId(i)).omega;
        vNL(i) = abs(switchboard(gensetSwbId(i)).voltage);
    end
end

== matlab function drillingRigMss/Central/Electric voltage calculations/Busses/Merge loads ==
  data: load input; loads output Bus: powerLoadsBus; swb2bus input
function loads  = mergeloads(load,swb2bus)
%#codegen
loads = repmat( struct( 'p',0,'q',0,'SwitchboardID',0),length(swb2bus),1);
for i = 1:length(load)
    bus = swb2bus(load(i).SwitchboardID);
    loads(bus).p = loads(bus).p+ load(i).p;
    loads(bus).q = loads(bus).q+ load(i).q;
end
for i = 1:length(swb2bus)
    loads(i).SwitchboardID = i;
end

== matlab function drillingRigMss/Controller/Embedded MATLAB Function2 ==
  data: y input; tau input; tauRt output
function tauRt = fcn(y,tau)
%#eml

Psi = y(3);

R = [cos(Psi) sin(Psi) 0;
   -sin(Psi)  cos(Psi) 0;
       0        0      1];
    
tauRt = R*tau;

== matlab function drillingRigMss/Controller/Embedded MATLAB Function3 ==
  data: y input; tau input; tauRt output
function tauRt = fcn(y,tau)
%#eml

Psi = y(3);

R = [cos(Psi) sin(Psi) 0;
   -sin(Psi)  cos(Psi) 0;
       0        0      1];
    
tauRt = R*tau;

== matlab function drillingRigMss/Central/Electric voltage calculations/Switchboard2Bus/MATLAB Function ==
  data: breaker input; nbus output size=1; nSwitchboards parameter size=1; switchboard2bus output size=nSwitchboards
function [nbus, switchboard2bus] = breaker2bus(breaker,nSwitchboards)
%#codegen
    switchboard2bus = (1:nSwitchboards)';
    for i = 1:length(breaker)
        if (breaker(i).BreakerStatus)
            swb1 = breaker(i).Swb1;
            swb2 = breaker(i).Swb2;
            busId1 = switchboard2bus(swb1);
            busId2 = switchboard2bus(swb2);
            busId = min(busId1,busId2);
            switchboard2bus(swb1) = busId;
            switchboard2bus(swb2) = busId;
        end
    end
    
nbus = 0;

for i = 1:nSwitchboards
   if switchboard2bus(i) == i;
       nbus = nbus +1;
       switchboard2bus(i) = nbus;
   else 
       switchboard2bus(i) = switchboard2bus(switchboard2bus(i));
   end
end

end

== matlab function drillingRigMss/Central/Electric voltage calculations/Busses/Thevenin Equivalent ==
  data: nbus input; switchboard2bus input; generatorset input; theveninEquivalent output Bus: TheveninBus
function theveninEquivalent  = mergeGenerators(nbus,switchboard2bus,generatorset)
%#codegen
nSwitchboards = length(switchboard2bus);
assert(nbus<=nSwitchboards);
nGeneratorset = length(generatorset);
E = complex(zeros(nGeneratorset,1));
Z = complex(zeros(nGeneratorset,1));
Sb = zeros(nGeneratorset,1);
Connected = zeros(nGeneratorset,1);
omega = zeros(nGeneratorset,1);
genset2swb = zeros(nGeneratorset,1);
for i = 1:nGeneratorset
    E(i) = generatorset(i).E;
    Z(i) = generatorset(i).Z;
    Sb(i) = generatorset(i).Sb;
    Connected(i) = generatorset(i).Connected;
    omega(i) = generatorset(i).omega;
    genset2swb(i) = generatorset(i).SwitchboardID;
end   

theveninEquivalent = repmat( struct( 'E',1j,'Z',1j,'Sb',0,'Connected',true,'omega',0,'SwitchboardID',0),nSwitchboards);
for bus = 1:nbus
    %Find gensets connected to bus
    m = 0;  
    for i = 1:nGeneratorset
        if (switchboard2bus(genset2swb(i))==bus && Connected(i))
            m = m + 1;
        end
    end
    assert(m <= nGeneratorset);
    gensets = zeros(1,m);
    m = 0;    
    for i = 1:nGeneratorset
        if (switchboard2bus(genset2swb(i))==bus && Connected(i))
            m = m + 1;
            gensets(m) = i;
        end
    end
    [ et, zt, Sb_bus, ~, omegaAvgBus ] = TheveninEquivalent( E(gensets), Z(gensets), Sb(gensets), Connected(gensets), omega(gensets) );
    theveninEquivalent(bus).E = et;
    theveninEquivalent(bus).Z = zt;
    theveninEquivalent(bus).Sb = Sb_bus;
    theveninEquivalent(bus).Connected = true;
    theveninEquivalent(bus).omega = omegaAvgBus;
    theveninEquivalent(bus).SwitchboardID = bus;
end

== matlab function drillingRigMss/Controller/anglemap ==
  data: y input; yo output
function yo = anglemap(y)
Psi = y(3);
x = mod(Psi,2*pi);
if x > pi
    x = x - 2*pi;
end

yo = [y(1); y(2); x];

== matlab function drillingRigMss/Controller/Embedded MATLAB Function1 ==
  data: y input; tau input; tauRt output
function tauRt = fcn(y,tau)
%#eml

Psi = y(3);

R = [cos(Psi) sin(Psi) 0;
   -sin(Psi)  cos(Psi) 0;
       0        0      1];
    
tauRt = R*tau;

== matlab function drillingRigMss/Observer/Bias estimator/Embedded MATLAB Function ==
  data: y input size=3; b_hat input; bRt output
function bRt = fcn(y,b_hat)
%#eml

Psi = y(3);

R = [cos(Psi) sin(Psi) 0;
     -sin(Psi)  cos(Psi) 0;
        0        0      1];
    
bRt = R*b_hat;

== matlab function drillingRigMss/Observer/Embedded MATLAB Function ==
  data: y input; nu_hat input; nuR output
function nuR = fcn(y,nu_hat)
%#eml

Psi = y(3);

R = [cos(Psi) -sin(Psi) 0;
     sin(Psi)  cos(Psi) 0;
        0        0      1];
    
nuR = R*nu_hat;

== matlab function drillingRigMss/Observer/Embedded MATLAB Function1 ==
  data: y input; b_hat input; bRt output
function bRt = fcn(y,b_hat)
%#eml

Psi = y(3);

R = [cos(Psi) sin(Psi) 0;
     -sin(Psi)  cos(Psi) 0;
        0        0      1];
    
bRt = R*b_hat;

== matlab function drillingRigMss/Observer/anglemap ==
  data: y input; yo output
function yo = anglemap(y)
Psi = y(3);
x = mod(Psi,2*pi);
if x > pi
    x = x - 2*pi;
end

yo = [y(1); y(2); x];
